simulink model "LCA"  (R2022b)
settings: Solver=FixedStepDiscrete  StartTime=0.0  StopTime=10.0  FixedStep=0.01  RelTol=1e-3
settings Model: DataDictionary=Lane_Changing_Assistant.sldd  Creator=MAAM  LastModifiedBy=MAAM
settings OptimizationCC: DefaultParameterBehavior=Inlined  UseDivisionForNetSlopeComputation=on  GainParamInheritBuiltInType=on  UseFloatMulNetSlope=on  UseSpecifiedMinMax=on  InlineInvariantSignals=on  BitwiseOrLogicalOp=Bitwise operator  PassReuseOutputArgsAs=Individual arguments  ZeroExternalMemoryAtStartup=off  ZeroInternalMemoryAtStartup=off  NoFixptDivByZeroProtection=on  EfficientFloat2IntCast=on  LifeSpan=inf  OptimizeBlockOrder=speed  DifferentSizesBufferReuse=on  EfficientTunableParamExpr=on
settings DebuggingCC: SignalInfNanChecking=error  ReadBeforeWriteMsg=EnableAllAsError  WriteAfterWriteMsg=EnableAllAsError  WriteAfterReadMsg=EnableAllAsError  AlgebraicLoopMsg=error  ArtificialAlgebraicLoopMsg=error  SaveWithDisabledLinksMsg=error  SaveWithParameterizedLinksMsg=error  BlockPriorityViolationMsg=error  InheritedTsInSrcMsg=error  SingleTaskRateTransMsg=error  TasksWithSamePriorityMsg=error  SigSpecEnsureSampleTimeMsg=error  CheckMatrixSingularityMsg=error  IntegerOverflowMsg=error  ParameterUnderflowMsg=error  ParameterPrecisionLossMsg=error  ParameterTunabilityLossMsg=error  UnderSpecifiedDataTypeMsg=error  UnnecessaryDatatypeConvMsg=warning  VectorMatrixConversionMsg=error  SignalLabelMismatchMsg=error  UnconnectedInputMsg=error  UnconnectedOutputMsg=error  UnconnectedLineMsg=error  SFcnCompatibilityMsg=error  UniqueDataStoreMsg=error  BusObjectLabelMismatch=error  RootOutportRequireBusObject=error  AssertControl=DisableAll  ModelReferenceIOMsg=error  ModelReferenceVersionMismatchMessage=error  ModelReferenceIOMismatchMessage=error  UnknownTsInhSupMsg=error  StateNameClashWarn=warning  StrictBusMsg=ErrorOnBusTreatedAsVector  NonBusSignalsTreatedAsBus=error  SFUnusedDataAndEventsDiag=error  SFInvalidInputDataAccessInChartInitDiag=error  SFTransitionOutsideNaturalParentDiag=error  SFUnreachableExecutionPathDiag=error  SFUndirectedBroadcastEventsDiag=error  SFTransitionActionBeforeConditionDiag=error  SFTemporalDelaySmallerThanSampleTimeDiag=error  SFSelfTransitionDiag=error  SFExecutionAtInitializationDiag=error  IntegerSaturationMsg=error  VariantConditionMismatch=error
settings HardwareCC: ProdBitPerPointer=32  ProdBitPerSizeT=32  ProdBitPerPtrDiffT=32  ProdLargestAtomicInteger=Long  ProdLargestAtomicFloat=Double  ProdWordSize=32  ProdLongLongMode=on  ProdHWDeviceType=ARM Compatible->ARM Cortex-M
settings SFSimCC: CompileTimeRecursionLimit=0  EnableRuntimeRecursion=off  MATLABDynamicMemAlloc=off
settings RTWCC: Description=AUTOSAR  SystemTargetFile=autosar.tlc  GenCodeOnly=on  TemplateMakefile=ert_default_tmf  BuildConfiguration=Faster Runs
settings CodeAppCC: ForceParamTrailComments=on  IgnoreCustomStorageClasses=off  IgnoreTestpoints=on  OperatorAnnotations=on  SimulinkDataObjDesc=on  SFDataObjDesc=on  MATLABFcnDesc=on  CustomSymbolStrGlobalVar=rt$N$M  CustomSymbolStrType=$N$M  CustomSymbolStrFcn=$N$M$F  CustomSymbolStrMacro=$N$M  InsertBlockDesc=on  ReqsInCode=on
settings STFCustomTargetCC: TargetLangStandard=C99 (ISO)  UtilityFuncGeneration=Shared location  MultiwordLength=256  ParMdlRefBuildCompliant=on  CompOptLevelCompliant=on  IncludeMdlTerminateFcn=off  CombineOutputUpdateFcns=on  CombineSignalStateStructs=on  SuppressErrorStatus=on  ERTCustomFileBanners=on  SupportAbsoluteTime=off  PurelyIntegerCode=on  SupportNonFinite=off  SupportComplex=off  SupportContinuousTime=off  SupportNonInlinedSFcns=off  RemoveResetFunc=on  ParenthesesLevel=Standards  CastingMode=Standards  MATLABClassNameForMDSCustomization=Simulink.SoftwareTarget.ERTCustomization  AutosarCompliant=on  UseToolchainInfoCompliant=on  GenerateSharedConstants=off  LookupTableObjectStructAxisOrder=2,1,3,4,...  LUTObjectStructOrderEvenSpacing=Size,Table,Breakpoints  SystemTargetFile=autosar.tlc
settings ERTTargetCC: TargetLangStandard=C99 (ISO)  UtilityFuncGeneration=Shared location  ConcurrentExecutionCompliant=off  IncludeMdlTerminateFcn=off  CombineSignalStateStructs=on  SuppressErrorStatus=on  SupportAbsoluteTime=off  PurelyIntegerCode=on  SupportNonFinite=off  SupportComplex=off  ParenthesesLevel=Standards  CastingMode=Standards  ModelStepFunctionPrototypeControlCompliant=off  CPPClassGenCompliant=off  AutosarCompliant=on  GenerateSharedConstants=off  LookupTableObjectStructAxisOrder=2,1,3,4,...  LUTObjectStructOrderEvenSpacing=Size,Table,Breakpoints  InlinedParameterPlacement=NonHierarchical  ERTCustomFileTemplate=example_file_process.tlc  PreserveExpressionOrder=on  EnableSignedLeftShifts=off  EnableSignedRightShifts=off
settings ConfigComp: CovScope=ReferencedModels

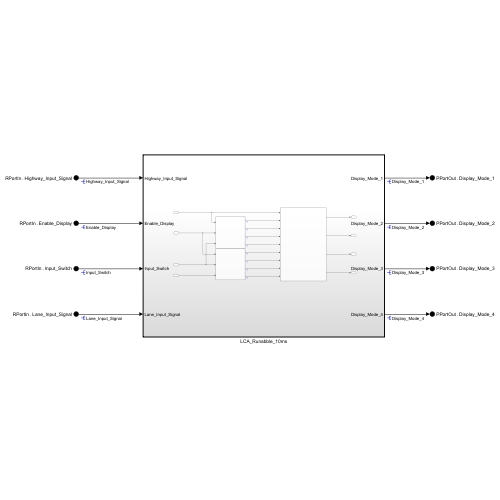
[thumbnail: Simulink's stored preview of the top-level diagram]
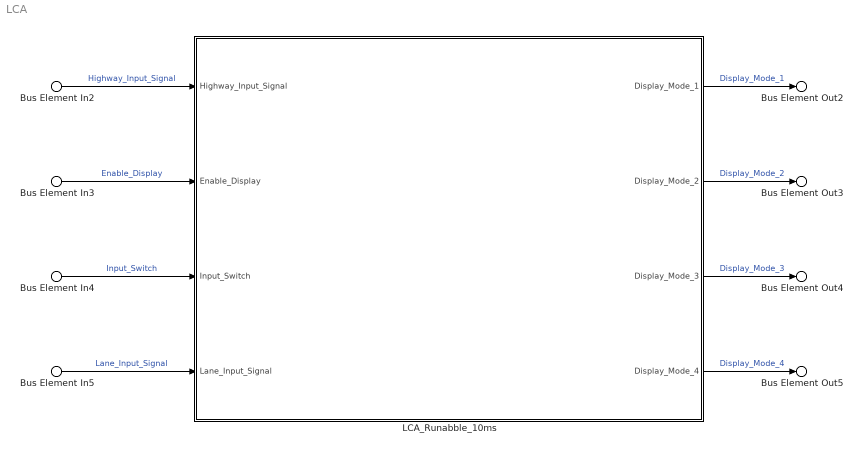
== system LCA ==
  Bus Element In2 : Inport  PortName=RPortIn  Element=Highway_Input_Signal
  Bus Element In5 : Inport  PortName=RPortIn  Element=Lane_Input_Signal
  Bus Element In4 : Inport  PortName=RPortIn  Element=Input_Switch
  Bus Element In3 : Inport  PortName=RPortIn  Element=Enable_Display
  LCA_Runabble_10ms : Subsystem  TreatAsAtomicUnit=on  SystemSampleTime=0.01
      settings: RTWSystemCode=Nonreusable function  RTWFcnNameOpts=Use subsystem name  RTWFileNameOpts=Use subsystem name  FunctionInterfaceSpec=Allow arguments (Optimized)
  Bus Element Out2 : Outport  PortName=PPortOut  Element=Display_Mode_1
  Bus Element Out3 : Outport  PortName=PPortOut  Element=Display_Mode_2
  Bus Element Out4 : Outport  PortName=PPortOut  Element=Display_Mode_3
  Bus Element Out5 : Outport  PortName=PPortOut  Element=Display_Mode_4
  wires:
  Bus Element In5/1 -> LCA_Runabble_10ms/4(Lane_Input_Signal)  "Lane_Input_Signal"
  Bus Element In4/1 -> LCA_Runabble_10ms/3(Input_Switch)  "Input_Switch"
  Bus Element In3/1 -> LCA_Runabble_10ms/2(Enable_Display)  "Enable_Display"
  Bus Element In2/1 -> LCA_Runabble_10ms/1(Highway_Input_Signal)  "Highway_Input_Signal"
  LCA_Runabble_10ms/4(Display_Mode_4) -> Bus Element Out5/1  "Display_Mode_4"
  LCA_Runabble_10ms/3(Display_Mode_3) -> Bus Element Out4/1  "Display_Mode_3"
  LCA_Runabble_10ms/2(Display_Mode_2) -> Bus Element Out3/1  "Display_Mode_2"
  LCA_Runabble_10ms/1(Display_Mode_1) -> Bus Element Out2/1  "Display_Mode_1"

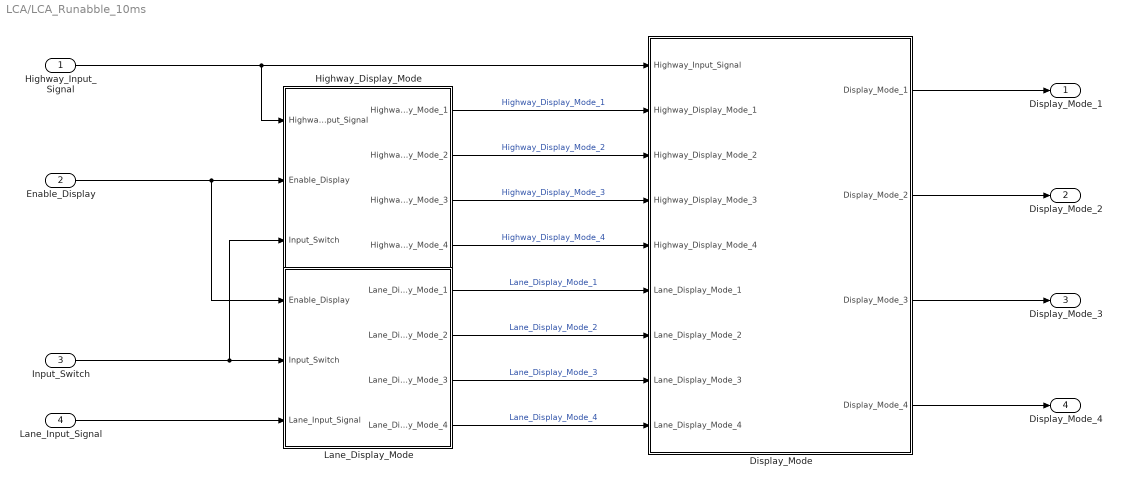
== system LCA/LCA_Runabble_10ms ==
  Highway_Input_Signal : Inport  OutDataTypeStr=uint8
  Enable_Display : Inport  Port=2  OutDataTypeStr=uint8
  Input_Switch : Inport  Port=3  OutDataTypeStr=uint8
  Lane_Input_Signal : Inport  Port=4  OutDataTypeStr=uint8
  Display_Mode : Subsystem
  Highway_Display_Mode : Subsystem
  Lane_Display_Mode : Subsystem
  Display_Mode_1 : Outport  OutDataTypeStr=uint8
  Display_Mode_2 : Outport  Port=2  OutDataTypeStr=uint8
  Display_Mode_3 : Outport  Port=3  OutDataTypeStr=uint8
  Display_Mode_4 : Outport  Port=4  OutDataTypeStr=uint8
  wires:
  Highway_Display_Mode/3(Highway_Display_Mode_3) -> Display_Mode/4(Highway_Display_Mode_3)  "Highway_Display_Mode_3"
  Lane_Display_Mode/3(Lane_Display_Mode_3) -> Display_Mode/8(Lane_Display_Mode_3)  "Lane_Display_Mode_3"
  Highway_Display_Mode/1(Highway_Display_Mode_1) -> Display_Mode/2(Highway_Display_Mode_1)  "Highway_Display_Mode_1"
  Lane_Display_Mode/4(Lane_Display_Mode_4) -> Display_Mode/9(Lane_Display_Mode_4)  "Lane_Display_Mode_4"
  Highway_Display_Mode/2(Highway_Display_Mode_2) -> Display_Mode/3(Highway_Display_Mode_2)  "Highway_Display_Mode_2"
  Input_Switch/1 -> Highway_Display_Mode/3(Input_Switch), Lane_Display_Mode/2(Input_Switch)
  Lane_Display_Mode/1(Lane_Display_Mode_1) -> Display_Mode/6(Lane_Display_Mode_1)  "Lane_Display_Mode_1"
  Enable_Display/1 -> Lane_Display_Mode/1(Enable_Display), Highway_Display_Mode/2(Enable_Display)
  Lane_Display_Mode/2(Lane_Display_Mode_2) -> Display_Mode/7(Lane_Display_Mode_2)  "Lane_Display_Mode_2"
  Lane_Input_Signal/1 -> Lane_Display_Mode/3(Lane_Input_Signal)
  Highway_Display_Mode/4(Highway_Display_Mode_4) -> Display_Mode/5(Highway_Display_Mode_4)  "Highway_Display_Mode_4"
  Highway_Input_Signal/1 -> Highway_Display_Mode/1(Highway_Input_Signal), Display_Mode/1(Highway_Input_Signal)
  Display_Mode/4(Display_Mode_4) -> Display_Mode_4/1
  Display_Mode/3(Display_Mode_3) -> Display_Mode_3/1
  Display_Mode/2(Display_Mode_2) -> Display_Mode_2/1
  Display_Mode/1(Display_Mode_1) -> Display_Mode_1/1

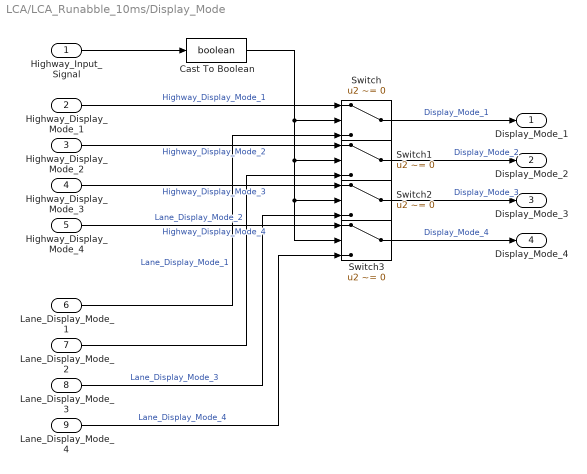
== system LCA/LCA_Runabble_10ms/Display_Mode ==
  Highway_Input_Signal : Inport
  Highway_Display_Mode_1 : Inport  Port=2  OutDataTypeStr=uint8
  Highway_Display_Mode_2 : Inport  Port=3  OutDataTypeStr=uint8
  Highway_Display_Mode_3 : Inport  Port=4  OutDataTypeStr=uint8
  Highway_Display_Mode_4 : Inport  Port=5  OutDataTypeStr=uint8
  Lane_Display_Mode_1 : Inport  Port=6  OutDataTypeStr=uint8
  Lane_Display_Mode_2 : Inport  Port=7  OutDataTypeStr=uint8
  Lane_Display_Mode_3 : Inport  Port=8  OutDataTypeStr=uint8
  Lane_Display_Mode_4 : Inport  Port=9  OutDataTypeStr=uint8
  Cast To Boolean : DataTypeConversion  OutDataTypeStr=boolean  SaturateOnIntegerOverflow=off  RndMeth=Floor
  Switch{,1..3} (4 alike) : Switch  Criteria=u2 ~= 0  OutDataTypeStr=Inherit: Inherit via back propagation  SaturateOnIntegerOverflow=off  InputSameDT=off
  Display_Mode_1 : Outport  OutDataTypeStr=uint8
  Display_Mode_2 : Outport  Port=2  OutDataTypeStr=uint8
  Display_Mode_3 : Outport  Port=3  OutDataTypeStr=uint8
  Display_Mode_4 : Outport  Port=4  OutDataTypeStr=uint8
  wires:
  Highway_Display_Mode_1/1 -> Switch/1  "Highway_Display_Mode_1"
  Highway_Display_Mode_2/1 -> Switch1/1  "Highway_Display_Mode_2"
  Highway_Display_Mode_3/1 -> Switch2/1  "Highway_Display_Mode_3"
  Highway_Display_Mode_4/1 -> Switch3/1  "Highway_Display_Mode_4"
  Lane_Display_Mode_1/1 -> Switch/3  "Lane_Display_Mode_1"
  Lane_Display_Mode_2/1 -> Switch1/3  "Lane_Display_Mode_2"
  Lane_Display_Mode_3/1 -> Switch2/3  "Lane_Display_Mode_3"
  Lane_Display_Mode_4/1 -> Switch3/3  "Lane_Display_Mode_4"
  Highway_Input_Signal/1 -> Cast To Boolean/1
  Switch/1 -> Display_Mode_1/1  "Display_Mode_1"
  Switch1/1 -> Display_Mode_2/1  "Display_Mode_2"
  Switch2/1 -> Display_Mode_3/1  "Display_Mode_3"
  Cast To Boolean/1 -> Switch1/2, Switch2/2, Switch3/2, Switch/2
  Switch3/1 -> Display_Mode_4/1  "Display_Mode_4"

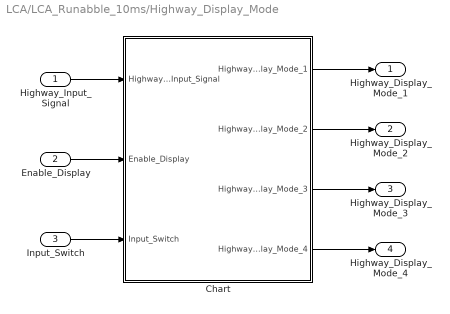
== system LCA/LCA_Runabble_10ms/Highway_Display_Mode ==
  Highway_Input_Signal : Inport  OutDataTypeStr=uint8
  Enable_Display : Inport  Port=2  OutDataTypeStr=uint8
  Input_Switch : Inport  Port=3  OutDataTypeStr=uint8
  Chart : Stateflow chart  TreatAsAtomicUnit=on
      settings: PortSchema="{\"entries\":[{\"content\":{\"sides\":[{\"content\":{\"connectorIds\":[\"In3\",\"In1\",\"In2\"]},\"type\":\"ConnectorPlacement.EquallySpacedRectSide\",\"uuid\":\"824ef089-422f-45fd-85ac-7da1f95e43cc\"},{\"content\":{\"connectorIds\":[\"Out1\",\"Out2\",\"Out3\",\"Out4\"],\"side\":\"RIGHT\"},\"type\":\"ConnectorPlacement.EquallySpacedRectSide\",\"uuid\":\"e93a6962-5bf9-412a-886e-d2082e9ef9b6\"},{\"content\":{\"connectorIds\":[],\"side\":\"TOP\"},\"type\":\"ConnectorPlacement.EquallySpacedRectSide\",\"uuid\":\"82451a30-e68f-46e9-9b96-50e6ee105f7a\"}]},\"type\":\"ConnectorPlacement.EquallySpacedConnector\",\"uuid\":\"ce25c2be-0560-41ec-a977-d6bde6a8128f\"}],\"packageUris\":[\"http://schema.mathworks.com/mf0/Connector/R2020b\"],\"version\":\"1.0\"}"
  Highway_Display_Mode_1 : Outport  OutDataTypeStr=uint8
  Highway_Display_Mode_2 : Outport  Port=2  OutDataTypeStr=uint8
  Highway_Display_Mode_3 : Outport  Port=3  OutDataTypeStr=uint8
  Highway_Display_Mode_4 : Outport  Port=4  OutDataTypeStr=uint8
  wires:
  Chart/1(Highway_Display_Mode_1) -> Highway_Display_Mode_1/1
  Chart/2(Highway_Display_Mode_2) -> Highway_Display_Mode_2/1
  Chart/3(Highway_Display_Mode_3) -> Highway_Display_Mode_3/1
  Chart/4(Highway_Display_Mode_4) -> Highway_Display_Mode_4/1
  Input_Switch/1 -> Chart/2(Input_Switch)
  Enable_Display/1 -> Chart/1(Enable_Display)
  Highway_Input_Signal/1 -> Chart/3(Highway_Input_Signal)

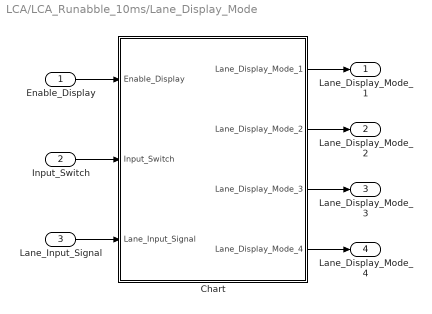
== system LCA/LCA_Runabble_10ms/Lane_Display_Mode ==
  Enable_Display : Inport  OutDataTypeStr=uint8
  Input_Switch : Inport  Port=2  OutDataTypeStr=uint8
  Lane_Input_Signal : Inport  Port=3  OutDataTypeStr=uint8
  Chart : Stateflow chart  TreatAsAtomicUnit=on
  Lane_Display_Mode_1 : Outport  OutDataTypeStr=uint8
  Lane_Display_Mode_2 : Outport  Port=2  OutDataTypeStr=uint8
  Lane_Display_Mode_3 : Outport  Port=3  OutDataTypeStr=uint8
  Lane_Display_Mode_4 : Outport  Port=4  OutDataTypeStr=uint8
  wires:
  Chart/4(Lane_Display_Mode_4) -> Lane_Display_Mode_4/1
  Chart/3(Lane_Display_Mode_3) -> Lane_Display_Mode_3/1
  Chart/2(Lane_Display_Mode_2) -> Lane_Display_Mode_2/1
  Chart/1(Lane_Display_Mode_1) -> Lane_Display_Mode_1/1
  Lane_Input_Signal/1 -> Chart/3(Lane_Input_Signal)
  Input_Switch/1 -> Chart/2(Input_Switch)
  Enable_Display/1 -> Chart/1(Enable_Display)

== stateflow chart LCA/LCA_Runabble_10ms/Lane_Display_Mode/Chart ==
  state TT_Logic [function]
    (default) -> (junction 50)
    (junction 50) -> (junction 52) : { aVarTruthTableCondition_1 = (Lane_Input_Signal == 6); }
    (junction 52) -> (junction 54) : { aVarTruthTableCondition_2 = (Enable_Display); }
    (junction 54) -> (junction 56) : { aVarTruthTableCondition_3 = (Input_Switch); }
    (junction 56) -> (junction 58) [order 1] : [!aVarTruthTableCondition_1]
    (junction 58) -> (junction 60) : {
        | /*  */
        |
        | }
    (junction 56) -> (junction 62) [order 2]
    (junction 62) -> (junction 64) [order 1] : [!aVarTruthTableCondition_3]
    (junction 64) -> (junction 66) : {
        | /*  */
        |
        | }
    (junction 62) -> (junction 68) [order 2]
    (junction 68) -> (junction 70) [order 1] : [aVarTruthTableCondition_1 && aVarTruthTableCondition_2 && aVarTruthTableCondition_3]
    (junction 70) -> (junction 72) : {
        | /*  */
        | Lane_Display_Mode_1 = 127
        | Lane_Display_Mode_2 = 248
        | Lane_Display_Mode_3 = 186
        | Lane_Display_Mode_4 = 84
        | }
    (junction 68) -> (junction 74) [order 2]
    (junction 74) -> (junction 76) : [aVarTruthTableCondition_1 && !aVarTruthTableCondition_2 && aVarTruthTableCondition_3]
    (junction 76) -> (junction 78) : {
        | /*  */
        | Lane_Display_Mode_1 = 132
        | Lane_Display_Mode_2 = 185
        | Lane_Display_Mode_3 = 54
        | Lane_Display_Mode_4 = 67
        | }
  state Run [parallel]
    en,du:
    TT_Logic();
    settings: executionOrder=1
  data: aVarTruthTableCondition_1 temporary boolean =0; aVarTruthTableCondition_2 temporary boolean =0; aVarTruthTableCondition_3 temporary boolean =0; Enable_Display input uint8; Lane_Display_Mode_1 output uint8; Lane_Display_Mode_2 output uint8; Lane_Display_Mode_3 output uint8; Lane_Display_Mode_4 output uint8; Input_Switch input uint8; Lane_Input_Signal input uint8

== stateflow chart LCA/LCA_Runabble_10ms/Highway_Display_Mode/Chart ==
  state TT_Logic [function]
    (junction 41) -> (junction 47) [order 2]
    (default) -> (junction 17)
    (junction 17) -> (junction 19) : { aVarTruthTableCondition_1 = (Highway_Input_Signal == 1); }
    (junction 19) -> (junction 21) : { aVarTruthTableCondition_2 = (Enable_Display); }
    (junction 21) -> (junction 23) : { aVarTruthTableCondition_3 = (Input_Switch); }
    (junction 23) -> (junction 25) [order 1] : [!aVarTruthTableCondition_1]
    (junction 25) -> (junction 27) : {  }
    (junction 23) -> (junction 29) [order 2]
    (junction 29) -> (junction 31) [order 1] : [!aVarTruthTableCondition_3]
    (junction 31) -> (junction 33) : {  }
    (junction 29) -> (junction 35) [order 2]
    (junction 35) -> (junction 37) [order 1] : [aVarTruthTableCondition_1 && aVarTruthTableCondition_2 && aVarTruthTableCondition_3]
    (junction 37) -> (junction 39) : {
        | Highway_Display_Mode_1 = 213
        | Highway_Display_Mode_2 = 183
        | Highway_Display_Mode_3 = 9
        | Highway_Display_Mode_4 = 94
        | }
    (junction 35) -> (junction 41) [order 2]
    (junction 41) -> (junction 43) [order 1] : [aVarTruthTableCondition_1 && !aVarTruthTableCondition_2 && aVarTruthTableCondition_3]
    (junction 43) -> (junction 45) : {
        | Highway_Display_Mode_1 = 232
        | Highway_Display_Mode_2 = 183
        | Highway_Display_Mode_3 = 41
        | Highway_Display_Mode_4 = 94
        | }
  state Run [parallel]
    en,du:
    TT_Logic();
    settings: executionOrder=1
  data: aVarTruthTableCondition_1 temporary boolean =0; aVarTruthTableCondition_2 temporary boolean =0; aVarTruthTableCondition_3 temporary boolean =0; Enable_Display input uint8; Highway_Display_Mode_1 output uint8; Highway_Display_Mode_2 output uint8; Highway_Display_Mode_3 output uint8; Highway_Display_Mode_4 output uint8; Input_Switch input uint8; Highway_Input_Signal input uint8
